simulink model "intentoFM"  (R2019a)
settings: Solver=VariableStepAuto  StartTime=0.0  StopTime=1  RelTol=1e-3
settings Model: Creator=JORGE  LastModifiedBy=JORGE

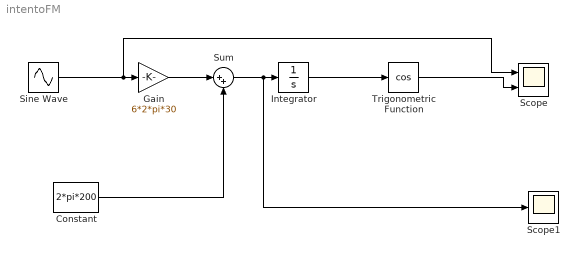
== system intentoFM ==
  Constant : Constant  Value=2*pi*200
  Gain : Gain  Gain=6*2*pi*30
  Integrator : Integrator
  Scope : Scope  NumInputPorts=2
  Scope1 : Scope
  Sine Wave : Sin  Frequency=2*pi*30  Phase=pi/2  SampleTime=1/10000
  Sum : Sum  Inputs=|++
  Trigonometric Function : Trigonometry  Operator=cos
  wires:
  Integrator/1 -> Trigonometric Function/1
  Sine Wave/1 -> Scope/1, Gain/1
  Gain/1 -> Sum/1
  Sum/1 -> Scope1/1, Integrator/1
  Trigonometric Function/1 -> Scope/2
  Constant/1 -> Sum/2
